simulink model "PLLtest"  (R2016a)
settings: Solver=VariableStepAuto  StartTime=0.0  StopTime=10.0  RelTol=1e-3
libraries: dspfdesign x1, dspsigops x1, dspsrcs4 x1
settings Model: Creator=lenovo  LastModifiedBy=lenovo

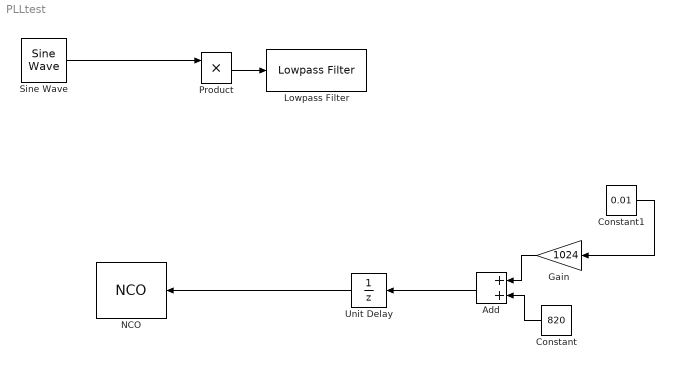
== system PLLtest ==
  Add : Sum  OutDataTypeStr=int16
  Constant : Constant  Value=820  OutDataTypeStr=int16  SampleTime=1/(8*10e5)
  Constant1 : Constant  Value=0.01  OutDataTypeStr=single  SampleTime=1/800000  LockScale=on
  Gain : Gain  Gain=1024  OutDataTypeStr=int16
  Lowpass Filter : dspfdesign/Lowpass Filter  FilterType=FIR  DesignForMinimumOrder=on  FilterOrder=50  PassbandFrequency=4*10e4  StopbandFrequency=8*10e4  PassbandRipple=0.1  StopbandAttenuation=80  InheritSampleRate=on  SampleRate=44100  roundingMode=Floor  coeffsDataTypeStr=fixdt(1,16)  SimulateUsing=Interpreted execution
  NCO : dspsigops/NCO  AccIncSrc=Input port  AccInc=100  PhaseOffsetSrc=Specify via dialog  PhaseOffset=0  AccumWL=16  HasDither=on  DitherWL=4  PNgeneratorLength=19  HasPhaseQuantizer=on  TableDepth=12  HasOutputPhaseError=off  Formula=Sine  DataType=single  OutputWL=16  OutputFL=14  CompMethod=Table lookup (no interpolation)  SampleTime=1  SamplesPerFrame=1  OutputFrames=off
  Product : Product
  Sine Wave : dspsrcs4/Sine Wave  Amplitude=1  Frequency=100  Phase=0  SampleMode=Discrete  OutComplex=Real  CompMethod=Trigonometric fcn  TableSize=Speed  SampleTime=1/800000  SamplesPerFrame=1  ResetState=Restart at time zero  OutputFrames=off  dataType=single  wordLen=16  udDataType=sfix(16)  fracBitsMode=Best precision  numFracBits=15  OutDataTypeStr=single  LastOutDataTypeStr=single
  Unit Delay : UnitDelay  SampleTime=-1
  wires:
  Sine Wave/1 -> Product/1
  Constant/1 -> Add/2
  Add/1 -> Unit Delay/1
  Unit Delay/1 -> NCO/1
  Product/1 -> Lowpass Filter/1
  Constant1/1 -> Gain/1
  Gain/1 -> Add/1
